simulink model "sarzni_reaktor"  (R2019b)
settings: Solver=ode45  StartTime=0.0  StopTime=40000  MaxStep=2  RelTol=1e-3  EnableMultiTasking=on
libraries: simulink x1
settings Model: Creator=Saso  LastModifiedBy=bonce
settings DataIOCC: LimitDataPoints=on  SaveFormat=Array  SignalLoggingSaveFormat=ModelDataLogs  SaveOutput=off  SignalLogging=off  DSMLogging=off
settings OptimizationCC: ExpressionDepthLimit=2147483647  InitFltsAndDblsToZero=on  LifeSpan=inf
settings DebuggingCC: SaveWithParameterizedLinksMsg=none  UnderspecifiedInitializationDetection=Classic  MergeDetectMultiDrivingBlocksExec=none  SignalResolutionControl=TryResolveAllWithWarning  SolverPrmCheckMsg=warning  MultiTaskDSMMsg=warning  MultiTaskCondExecSysMsg=none  FcnCallInpInsideContextMsg=warning  StateNameClashWarn=warning  SFUnexpectedBacktrackingDiag=warning  SFNoUnconditionalDefaultTransitionDiag=warning  SFExecutionAtInitializationDiag=none  ArithmeticOperatorsInVariantConditions=warning
settings HardwareCC: ProdBitPerPointer=32  ProdBitPerSizeT=32  ProdBitPerPtrDiffT=32  ProdLargestAtomicFloat=None  ProdIntDivRoundTo=Undefined  ProdEndianess=Unspecified  ProdWordSize=32  ProdHWDeviceType=32-bit Generic
settings ModelReferenceCC: PropagateSignalLabelsOutOfModel=off
settings SFSimCC: SimUseLocalCustomCode=off  CustomCodeUndefinedFunction=UseInterfaceOnly
settings RTWCC: RTWUseLocalCustomCode=off
settings CodeAppCC: StateflowObjectComments=on
settings GRTTargetCC: TargetFcnLib=ansi_tfl_tmw.mat  TargetLangStandard=C89/C90 (ANSI)  CombineOutputUpdateFcns=off  GRTInterface=on
settings ConfigComp: CovMetricSettings=dw  CovHtmlReporting=on  CovSaveCumulativeToWorkspaceVar=on  CovSaveSingleToWorkspaceVar=on  CovExternalEMLEnable=off

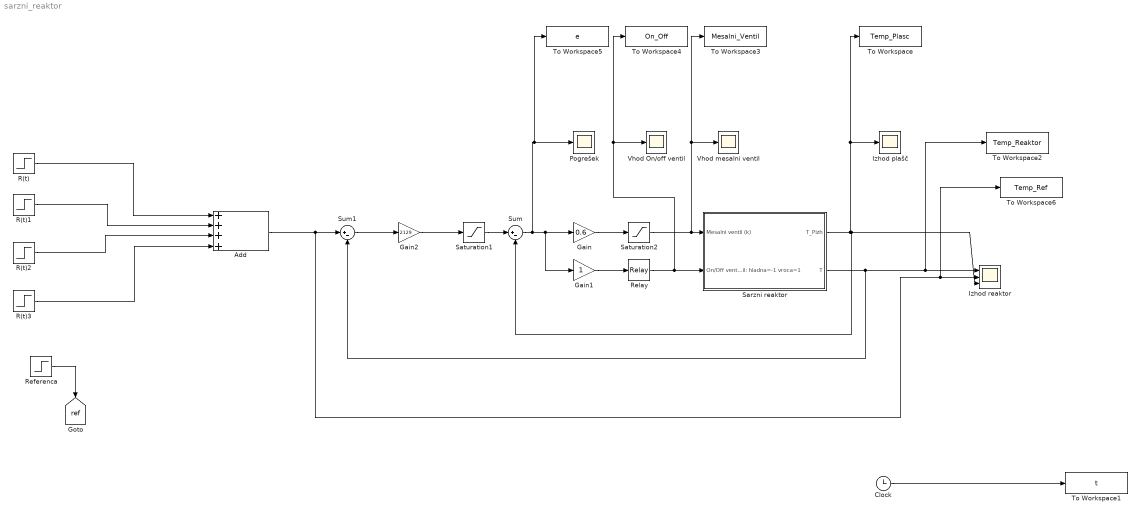
== system sarzni_reaktor ==
  Add : Sum  Inputs=4
  Clock : Clock
  Gain : Gain  Gain=0.6
  Gain1 : Gain
  Gain2 : Gain  Gain=2129
  Izhod plašč : Scope
  Izhod reaktor : Scope  NumInputPorts=3
  Pogrešek : Scope
  R(t) : Step  Time=0  Before=17  After=52  SampleTime=0
  R(t)1 : Step  Time=10000  After=-6  SampleTime=0
  R(t)2 : Step  Time=15000  After=4  SampleTime=0
  R(t)3 : Step  Time=20000  After=-17  SampleTime=0
  Referenca : Step  Time=10000  Before=40  After=45  SampleTime=0
  Relay : Relay  OnSwitchValue=0.1  OffSwitchValue=-0.1  OffOutputValue=-1
  Sarzni reaktor : Subsystem  mask(Sarzni reaktor){anim=0, sum=off}
      mask prompts: anim "Perioda vzorcenja animacije ali 0 (brez animacije)"; sum "Omogoci merilni sum"
      mask help: Sarzni reaktor.
      mask init:
      | T0 = 17; % Temperatura okolice
      | TH = 12; % Temperatura hladne vode
      | TV = 75; % Temperatura vroce vode
      | fiP = 1.6; % Masni pretok tekocine skozi plasc
      | m = 600; % Masa snovi v kotlu
      | mP = 40; % Masa snovi v plascu
      | lambda = 420; % Toplotna prevodnost spoja med plascem in kotlom
      | lambda0 = 84; % Toplotna prevodnost spoja med plascem in okolico
      | S = 2; % Skupna povrsina spoja med plascem in kotlom
      | S0 = 2; % Skupna povrsina spoja med plascem in okolico
      | cP = 4200; % Specificna toplota snovi v plascu
      | c = 4200; % Specificna toplota snovi v kotlu
      | 
      | TPizh_start = T0; % Zacetna izhodna temperatura plasca
      | T_start = T0; % Zacetna temperatura snovi v kotlu
      | 
      | varT = 0.01; % Merilni sum
      | Ts = 1; % Perioda vzorcenja meritev
  Saturation1 : Saturate  UpperLimit=60  LowerLimit=10
  Saturation2 : Saturate  UpperLimit=1  LowerLimit=0
  Sum : Sum  Inputs=|+-
  Sum1 : Sum  Inputs=|+-
  To Workspace : ToWorkspace  VariableName=Temp_Plasc  SampleTime=-1
  To Workspace1 : ToWorkspace  VariableName=t  SampleTime=-1
  To Workspace2 : ToWorkspace  VariableName=Temp_Reaktor  SampleTime=-1
  To Workspace3 : ToWorkspace  VariableName=Mesalni_Ventil  SampleTime=-1
  To Workspace4 : ToWorkspace  VariableName=On_Off  SampleTime=-1
  To Workspace5 : ToWorkspace  VariableName=e  SampleTime=-1
  To Workspace6 : ToWorkspace  VariableName=Temp_Ref  SampleTime=-1
  Vhod On/off ventil : Scope
  Vhod mesalni ventil : Scope
  tag scope: ref=global
  wires:
  Referenca/1 -> [ref]
  R(t)1/1 -> Add/2
  R(t)3/1 -> Add/4
  R(t)2/1 -> Add/3
  R(t)/1 -> Add/1
  Gain/1 -> Saturation2/1
  Sum/1 -> To Workspace5/1, Pogrešek/1, Gain1/1, Gain/1
  Sarzni reaktor/1(T_Pizh) -> Izhod reaktor/3, Sum/2, Izhod plašč/1, To Workspace/1
  Relay/1 -> Vhod On/off ventil/1, To Workspace4/1, Sarzni reaktor/2(On/Off ventil: hladna=-1 vroca=1)
  Gain1/1 -> Relay/1
  Saturation1/1 -> Sum/1
  Sarzni reaktor/2(T) -> To Workspace2/1, Izhod reaktor/1, Sum1/2
  Sum1/1 -> Gain2/1
  Gain2/1 -> Saturation1/1
  Add/1 -> To Workspace6/1, Izhod reaktor/2, Sum1/1
  Clock/1 -> To Workspace1/1
  Saturation2/1 -> To Workspace3/1, Vhod mesalni ventil/1, Sarzni reaktor/1(Mesalni ventil (k))

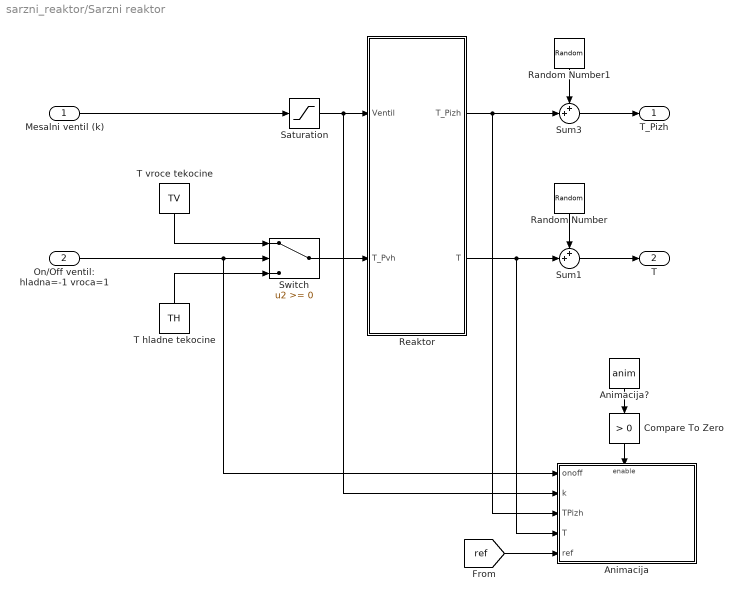
== system sarzni_reaktor/Sarzni reaktor ==
  Mesalni ventil (k) : Inport
  On/Off ventil: hladna=-1 vroca=1 : Inport  Port=2
  Animacija : Subsystem
  Animacija? : Constant  Value=anim
  Compare To Zero : simulink/Logic and Bit Operations/Compare To Zero  relop=>  OutDataTypeStr=boolean  ZeroCross=off
  Random Number : RandomNumber  Variance=varT*sum  Seed=round(rand*10000)  SampleTime=Ts*sum
  Random Number1 : RandomNumber  Variance=varT*sum  Seed=round(rand*10000)  SampleTime=Ts*sum
  Reaktor : Subsystem
  Saturation : Saturate  UpperLimit=1  LowerLimit=0
  Sum1 : Sum  Inputs=++|
  Sum3 : Sum  Inputs=++|
  Switch : Switch
  T hladne tekocine : Constant  Value=TH
  T vroce tekocine : Constant  Value=TV
  T_Pizh : Outport
  T : Outport  Port=2
  wires:
  Saturation/1 -> Animacija/2(k), Reaktor/1(Ventil)
  On/Off ventil: hladna=-1 vroca=1/1 -> Animacija/1(onoff), Switch/2
  T vroce tekocine/1 -> Switch/1
  T hladne tekocine/1 -> Switch/3
  Switch/1 -> Reaktor/2(T_Pvh)
  Sum3/1 -> T_Pizh/1
  Sum1/1 -> T/1
  Random Number/1 -> Sum1/1
  Random Number1/1 -> Sum3/1
  Mesalni ventil (k)/1 -> Saturation/1
  Reaktor/1(T_Pizh) -> Sum3/2, Animacija/3(TPizh)
  Reaktor/2(T) -> Sum1/2, Animacija/4(T)
  [ref] -> Animacija/5(ref)
  Animacija?/1 -> Compare To Zero/1
  Compare To Zero/1 -> Animacija/Enable

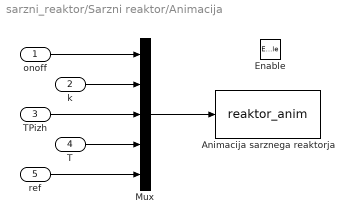
== system sarzni_reaktor/Sarzni reaktor/Animacija ==
  onoff : Inport
  k : Inport  Port=2
  TPizh : Inport  Port=3
  T : Inport  Port=4
  ref : Inport  Port=5
  Enable : EnablePort
  Animacija sarznega reaktorja : S-Function  FunctionName=reaktor_anim  Parameters=anim  SFunctionDeploymentMode=off  EnableBusSupport=off
  Mux : Mux  Inputs=5
  wires:
  ref/1 -> Mux/5
  T/1 -> Mux/4
  onoff/1 -> Mux/1
  Mux/1 -> Animacija sarznega reaktorja/1
  TPizh/1 -> Mux/3
  k/1 -> Mux/2

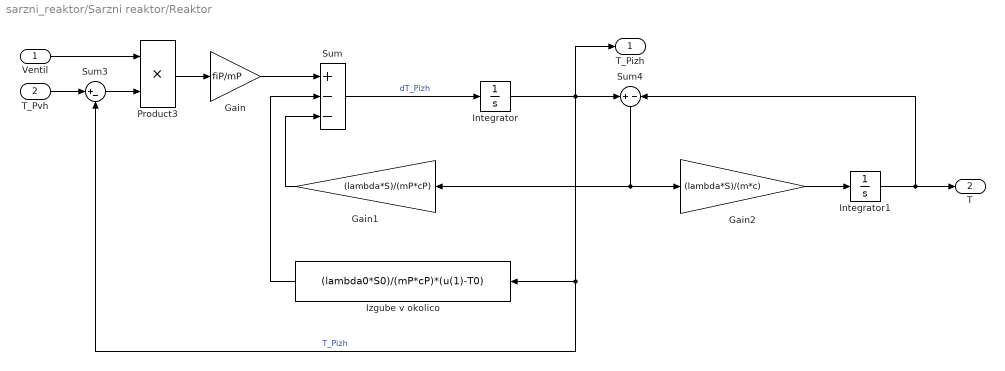
== system sarzni_reaktor/Sarzni reaktor/Reaktor ==
  Ventil : Inport
  T_Pvh : Inport  Port=2
  Gain : Gain  Gain=fiP/mP
  Gain1 : Gain  Gain=(lambda*S)/(mP*cP)
  Gain2 : Gain  Gain=(lambda*S)/(m*c)  SaturateOnIntegerOverflow=on  OutDataTypeStr=Inherit: Same as input  ParamDataTypeStr=Inherit: Same as input
  Integrator : Integrator  InitialCondition=TPizh_start
  Integrator1 : Integrator  InitialCondition=T_start
  Izgube v okolico : Fcn  Expr=(lambda0*S0)/(mP*cP)*(u(1)-T0)
  Product3 : Product  SaturateOnIntegerOverflow=on  RndMeth=Zero  InputSameDT=on  OutDataTypeStr=Inherit: Same as first input
  Sum : Sum  Inputs=+--  SaturateOnIntegerOverflow=on  InputSameDT=on  OutDataTypeStr=Inherit: Same as first input
  Sum3 : Sum  Inputs=|+-
  Sum4 : Sum  Inputs=+|-
  T_Pizh : Outport
  T : Outport  Port=2
  wires:
  Izgube v okolico/1 -> Sum/2
  Integrator/1 -> Sum3/2, Izgube v okolico/1, Sum4/1, T_Pizh/1  "T_Pizh"
  Sum/1 -> Integrator/1  "dT_Pizh"
  Product3/1 -> Gain/1
  Gain2/1 -> Integrator1/1
  Integrator1/1 -> T/1, Sum4/2
  T_Pvh/1 -> Sum3/1
  Gain/1 -> Sum/1
  Gain1/1 -> Sum/3
  Ventil/1 -> Product3/1
  Sum3/1 -> Product3/2
  Sum4/1 -> Gain1/1, Gain2/1
